simulink model "multi_ca_sim_1"  (R2020a)
settings: Solver=FixedStepAuto  StartTime=0.0  StopTime=23  FixedStep=0.01  MinStep=0.01  RelTol=1e-3
values from neighbouring files (symbols this model uses):
  ar_max = beta^2*omega/gamma/pi*0.999    (= 2.172825)    [SimulationSetup.m]
  beta = pi/tau_r    (= 3.14159265359)    [SimulationSetup.m]
  gamma = tau_r*beta + pi    (= 6.28318530718)    [SimulationSetup.m]
  Gamma = 10    [SimulationSetup.m]
  k = (gamma/beta)^2*(vo_max*psio_max) +0.1    (= 0.235)    [SimulationSetup.m]
  k_1 = 0.2    [SimulationSetup.m]
  k_2 = gamma^2/beta    (= 12.5663706144)    [SimulationSetup.m]
  k_delta = 1    [SimulationSetup.m]
  omega = r + (vr_max + vo_max)*pi/beta +0.1    (= 4.35)    [SimulationSetup.m]
  r = 2.0    (= 2)    [SimulationSetup.m]
  theta_0_1 = 0    [SimulationSetup.m]
  theta_0_2 = 0    [SimulationSetup.m]
  theta_0_3 = 0    [SimulationSetup.m]
  theta_a = pi/4    (= 0.785398163397)    [SimulationSetup.m]
  u_ca_max = 10    [SimulationSetup.m]
  u_tr_max = min(beta,beta^2*omega/(vr_max*gamma))    [SimulationSetup.m]
  vo_max = 0.75    [SimulationSetup.m]
  vr_max = 1.5    [SimulationSetup.m]
  vr_min = 1.0    (= 1)    [SimulationSetup.m]
  x_F_0_1 = -6    [SimulationSetup.m]
  x_F_0_2 = -4    [SimulationSetup.m]
  x_F_0_3 = -5    [SimulationSetup.m]
  y_F_0_1 = 0    [SimulationSetup.m]
  y_F_0_2 = -2    [SimulationSetup.m]
  y_F_0_3 = -4    [SimulationSetup.m]
libraries: cstblocks x3, dspmathops x3
(part 1 of 2)
settings Model: Creator=thiagomarinho  LastModifiedBy=tcy98
settings DataIOCC: ReturnWorkspaceOutputs=off
settings DebuggingCC: ArithmeticOperatorsInVariantConditions=warning
settings SFSimCC: CustomCodeUndefinedFunction=UseInterfaceOnly

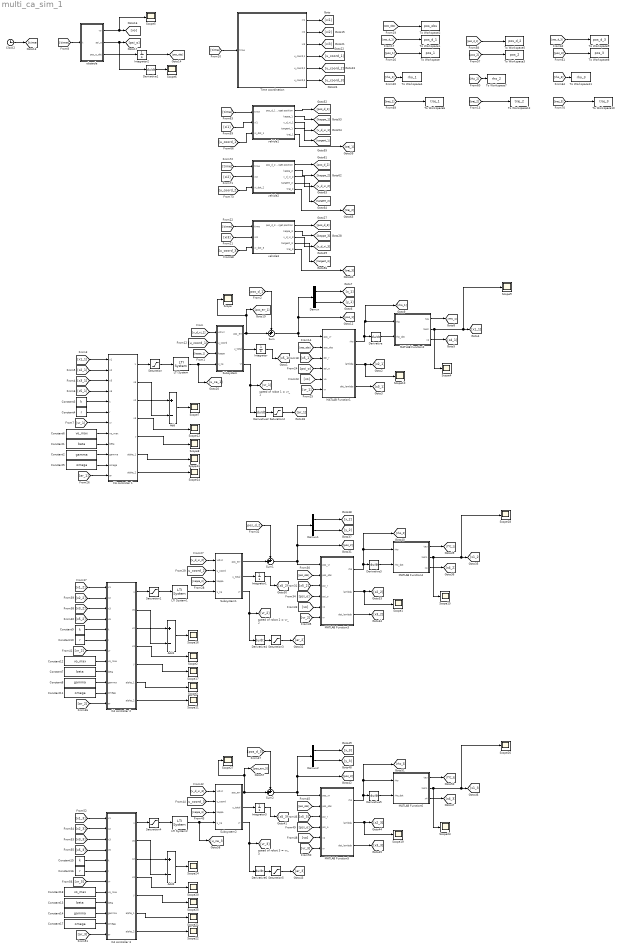
== system multi_ca_sim_1 ==
  Add : Sum  Inputs=+-
  Add1 : Sum  Inputs=+-
  Add2 : Sum  Inputs=+-
  CA controller 1 : MATLAB Function  TreatAsAtomicUnit=on
  CA controller 2 : MATLAB Function  TreatAsAtomicUnit=on
  CA controller 3 : MATLAB Function  TreatAsAtomicUnit=on
  Clock2 : Clock
  Constant1 : Constant  Value=beta
  Constant10 : Constant  Value=r
  Constant11 : Constant  Value=omega
  Constant12 : Constant  Value=vo_max
  Constant13 : Constant  Value=beta
  Constant14 : Constant  Value=gamma
  Constant15 : Constant  Value=k
  Constant16 : Constant  Value=r
  Constant17 : Constant  Value=omega
  Constant18 : Constant  Value=vo_max
  Constant2 : Constant  Value=gamma
  Constant3 : Constant  Value=k
  Constant4 : Constant  Value=r
  Constant5 : Constant  Value=omega
  Constant6 : Constant  Value=vo_max
  Constant7 : Constant  Value=beta
  Constant8 : Constant  Value=gamma
  Constant9 : Constant  Value=k
  Demux : Demux  Outputs=2
  Demux1 : Demux  Outputs=2
  Demux2 : Demux  Outputs=2
  Derivative{,1..6} (7 alike) : Derivative  CoefficientInTFapproximation=500
  Integrator : Integrator
  Integrator1 : Integrator
  Integrator2 : Integrator  InitialCondition=[0 0]'
  Integrator3 : Integrator
  LTI System : cstblocks/LTI System  sys=tf(1,[1 1])  IC=[]
  LTI System1 : cstblocks/LTI System  sys=tf(1,[1 1])  IC=[]
  LTI System2 : cstblocks/LTI System  sys=tf(1,[1 1])  IC=[]
  MATLAB Function1 : MATLAB Function  TreatAsAtomicUnit=on
  MATLAB Function2 : MATLAB Function  TreatAsAtomicUnit=on
  MATLAB Function3 : MATLAB Function  TreatAsAtomicUnit=on
  MATLAB Function4 : MATLAB Function  TreatAsAtomicUnit=on
  MATLAB Function5 : MATLAB Function  TreatAsAtomicUnit=on
  MATLAB Function6 : MATLAB Function  TreatAsAtomicUnit=on
  Saturation : Saturate  UpperLimit=u_ca_max  LowerLimit=-u_ca_max
  Saturation1 : Saturate  UpperLimit=u_ca_max  LowerLimit=-u_ca_max
  Saturation2 : Saturate  UpperLimit=ar_max  LowerLimit=-ar_max
  Saturation3 : Saturate  UpperLimit=ar_max  LowerLimit=-ar_max
  Saturation4 : Saturate  UpperLimit=u_ca_max  LowerLimit=-u_ca_max
  Saturation5 : Saturate  UpperLimit=ar_max  LowerLimit=-ar_max
  Scope{,1..27} (28 alike) : Scope
  Subsystem : Subsystem
  Subsystem1 : Subsystem
  Subsystem2 : Subsystem
  Sum : Sum  Inputs=++|
  Sum1 : Sum  Inputs=++|
  Sum2 : Sum  Inputs=++|
  Time coordination : Subsystem
  To Workspace : ToWorkspace  VariableName=pos_1  SaveFormat=Structure With Time  SampleTime=-1
  To Workspace1 : ToWorkspace  VariableName=pos_d_1  SaveFormat=Structure With Time  SampleTime=-1
  To Workspace10 : ToWorkspace  VariableName=traj_3  SaveFormat=Timeseries  SampleTime=-1
  To Workspace11 : ToWorkspace  VariableName=rho_3  SaveFormat=Timeseries  SampleTime=-1
  To Workspace12 : ToWorkspace  VariableName=traj_2  SaveFormat=Timeseries  SampleTime=-1
  To Workspace2 : ToWorkspace  VariableName=pos_obs  SaveFormat=Structure With Time  SampleTime=-1
  To Workspace3 : ToWorkspace  VariableName=pos_2  SaveFormat=Structure With Time  SampleTime=-1
  To Workspace4 : ToWorkspace  VariableName=rho_1  SaveFormat=Timeseries  SampleTime=-1
  To Workspace5 : ToWorkspace  VariableName=pos_d_2  SaveFormat=Structure With Time  SampleTime=-1
  To Workspace6 : ToWorkspace  VariableName=traj_1  SaveFormat=Timeseries  SampleTime=-1
  To Workspace7 : ToWorkspace  VariableName=rho_2  SaveFormat=Timeseries  SampleTime=-1
  To Workspace8 : ToWorkspace  VariableName=pos_3  SaveFormat=Structure With Time  SampleTime=-1
  To Workspace9 : ToWorkspace  VariableName=pos_d_3  SaveFormat=Structure With Time  SampleTime=-1
  obstacle : MATLAB Function  TreatAsAtomicUnit=on
  vehicle1 : Subsystem
  vehicle2 : Subsystem
  vehicle3 : Subsystem
  wires:
  obstacle/1(vo) -> Scope5/1, [vo]
  obstacle/2(psi_o) -> Derivative1/1, [psi_o]
  Integrator2/1 -> [pos_obs]
  obstacle/3(pos_o_dot) -> Integrator2/1
  Derivative1/1 -> Scope6/1
  [pos_obs] -> To Workspace2/1
  [pos_d_1] -> To Workspace1/1
  [v_d_xi_1] -> Subsystem/1(vd(xi))
  [kappa_1] -> Subsystem/3(kappa)
  [pos_d_1] -> Sum/1
  LTI System/1 -> [u_ca_1], Subsystem/4(u_ca)
  [pos_1] -> To Workspace/1
  MATLAB Function2/2(loom) -> Scope9/1, [x1_1], Scope4/1
  [vr_1] -> MATLAB Function1/6(vr)
  [x5_1] -> MATLAB Function1/3(psi_r)
  [vo] -> MATLAB Function1/5(vo)
  Demux/2 -> [y_1]
  MATLAB Function2/1(tau) -> [TTC_1]
  Derivative/1 -> MATLAB Function2/2(rho_dot)
  MATLAB Function2/3(x4) -> [x4_1]
  Demux/1 -> [x_1]
  MATLAB Function1/3(dot_lambda) -> [x3_1]
  [psi_o] -> MATLAB Function1/4(psi_o)
  MATLAB Function1/2(lambda) -> Scope10/1, [x2_1]
  [pos_obs] -> MATLAB Function1/2(pos_obs)
  MATLAB Function1/1(rho) -> [rho_1], MATLAB Function2/1(rho), Derivative/1
  CA controller 1/2(x5) -> Add/1
  CA controller 1/6(alpha_1) -> Scope13/1
  CA controller 1/5(y) -> Scope8/1
  [ar_1] -> CA controller 1/12(ar)
  [vr_1] -> CA controller 1/7(vr)
  CA controller 1/4(x3) -> Scope12/1
  CA controller 1/3(x2) -> Add/2
  Saturation/1 -> LTI System/1
  Constant5/1 -> CA controller 1/11(omega)
  Constant2/1 -> CA controller 1/10(gamma)
  CA controller 1/7(alpha_2) -> Scope14/1
  Constant1/1 -> CA controller 1/9(beta)
  Constant6/1 -> CA controller 1/8(vo_max)
  CA controller 1/1(u) -> Saturation/1
  Add/1 -> Scope7/1
  [x1_1] -> CA controller 1/1(x1)
  Constant3/1 -> CA controller 1/5(k)
  [x3_1] -> CA controller 1/3("x3 ")
  [x5_1] -> CA controller 1/4("x5 ")
  Constant4/1 -> CA controller 1/6(r)
  [x2_1] -> CA controller 1/2("x2 ")
  Subsystem/2(u_total) -> Integrator/1
  Integrator/1 -> [x5_1]
  Subsystem/3(vr) -> Derivative2/1, [vr_1]
  [rho_1] -> To Workspace4/1
  Saturation2/1 -> [ar_1]
  Derivative2/1 -> Saturation2/1
  Clock2/1 -> [time]
  [time] -> obstacle/1(t)
  [time] -> Time coordination/1(time)
  Sum/1 -> Demux/1, [pos_1], MATLAB Function1/1(pos_vr)
  Subsystem/1(pos_err) -> Sum/2, Scope/1, [pos_err_1]
  Time coordination/1(xi1) -> [xi1]
  Time coordination/2(xi2) -> [xi2]
  Time coordination/3(xi3) -> [xi3]
  Time coordination/4(u_coord,1) -> [u_coord_1]
  Time coordination/5(u_coord,2) -> [u_coord_2]
  Time coordination/6(u_coord,3) -> [u_coord_3]
  [u_coord_1] -> Subsystem/2(u_coord)
  [pos_d_2] -> Sum1/1
  Sum1/1 -> Demux1/1, [pos_2], MATLAB Function3/1(pos_vr)
  [x5_2] -> CA controller 2/4("x5 ")
  Constant10/1 -> CA controller 2/6(r)
  Constant7/1 -> CA controller 2/9(beta)
  Demux1/2 -> [y_2]
  [x5_2] -> MATLAB Function3/3(psi_r)
  Constant8/1 -> CA controller 2/10(gamma)
  Saturation1/1 -> LTI System1/1
  Constant12/1 -> CA controller 2/8(vo_max)
  [x2_2] -> CA controller 2/2("x2 ")
  Subsystem1/2(u_total) -> Integrator1/1
  CA controller 2/2(x5) -> Add1/1
  [pos_obs] -> MATLAB Function3/2(pos_obs)
  MATLAB Function3/3(dot_lambda) -> [x3_2]
  MATLAB Function3/2(lambda) -> Scope1/1, [x2_2]
  MATLAB Function3/1(rho) -> [rho_2], MATLAB Function4/1(rho), Derivative3/1
  CA controller 2/1(u) -> Saturation1/1
  [vr_2] -> CA controller 2/7(vr)
  [kappa_2] -> Subsystem1/3(kappa)
  [vo] -> MATLAB Function3/5(vo)
  [ar_2] -> CA controller 2/12(ar)
  Constant11/1 -> CA controller 2/11(omega)
  CA controller 2/5(y) -> Scope17/1
  [vr_2] -> MATLAB Function3/6(vr)
  MATLAB Function4/2(loom) -> Scope18/1, [x1_2], Scope15/1
  CA controller 2/3(x2) -> Add1/2
  Derivative3/1 -> MATLAB Function4/2(rho_dot)
  MATLAB Function4/1(tau) -> [TTC_2]
  MATLAB Function4/3(x4) -> [x4_2]
  Subsystem1/1(pos_err) -> Sum1/2
  Constant9/1 -> CA controller 2/5(k)
  [x3_2] -> CA controller 2/3("x3 ")
  Derivative4/1 -> Saturation3/1
  [x1_2] -> CA controller 2/1(x1)
  CA controller 2/7(alpha_2) -> Scope11/1
  Integrator1/1 -> [x5_2]
  Subsystem1/3(vr) -> Derivative4/1, [vr_2]
  [v_d_xi_2] -> Subsystem1/1(vd(xi))
  Add1/1 -> Scope16/1
  [psi_o] -> MATLAB Function3/4(psi_o)
  LTI System1/1 -> Subsystem1/4(u_ca)
  [u_coord_2] -> Subsystem1/2(u_coord)
  Saturation3/1 -> [ar_2]
  CA controller 2/6(alpha_1) -> Scope3/1
  CA controller 2/4(x3) -> Scope2/1
  Demux1/1 -> [x_2]
  [pos_d_3] -> Sum2/1
  Sum2/1 -> Demux2/1, [pos_3], MATLAB Function5/1(pos_vr)
  [x5_3] -> CA controller 3/4("x5 ")
  Constant16/1 -> CA controller 3/6(r)
  Constant13/1 -> CA controller 3/9(beta)
  Demux2/2 -> [y_3]
  [x5_3] -> MATLAB Function5/3(psi_r)
  Constant14/1 -> CA controller 3/10(gamma)
  Saturation4/1 -> LTI System2/1
  Constant18/1 -> CA controller 3/8(vo_max)
  [x2_3] -> CA controller 3/2("x2 ")
  Subsystem2/2(u_total) -> Integrator3/1
  CA controller 3/2(x5) -> Add2/1
  [pos_obs] -> MATLAB Function5/2(pos_obs)
  MATLAB Function5/3(dot_lambda) -> [x3_3]
  MATLAB Function5/2(lambda) -> Scope19/1, [x2_3]
  MATLAB Function5/1(rho) -> [rho_3], MATLAB Function6/1(rho), Derivative5/1
  CA controller 3/1(u) -> Saturation4/1
  [vr_3] -> CA controller 3/7(vr)
  [kappa_3] -> Subsystem2/3(kappa)
  [vo] -> MATLAB Function5/5(vo)
  [ar_3] -> CA controller 3/12(ar)
  Constant17/1 -> CA controller 3/11(omega)
  CA controller 3/5(y) -> Scope25/1
  [vr_3] -> MATLAB Function5/6(vr)
  MATLAB Function6/2(loom) -> Scope26/1, [x1_3], Scope23/1
  CA controller 3/3(x2) -> Add2/2
  Derivative5/1 -> MATLAB Function6/2(rho_dot)
  MATLAB Function6/1(tau) -> [TTC_3]
  MATLAB Function6/3(x4) -> [x4_3]
  Subsystem2/1(pos_err) -> Sum2/2, Scope27/1, [pos_err_3]
  Constant15/1 -> CA controller 3/5(k)
  [x3_3] -> CA controller 3/3("x3 ")
  Derivative6/1 -> Saturation5/1
  [x1_3] -> CA controller 3/1(x1)
  CA controller 3/7(alpha_2) -> Scope22/1
  Integrator3/1 -> [x5_3]
  Subsystem2/3(vr) -> Derivative6/1, [vr_3]
  [v_d_xi_3] -> Subsystem2/1(vd(xi))
  Add2/1 -> Scope24/1
  [psi_o] -> MATLAB Function5/4(psi_o)
  LTI System2/1 -> [u_ca_3], Subsystem2/4(u_ca)
  [u_coord_3] -> Subsystem2/2(u_coord)
  Saturation5/1 -> [ar_3]
  CA controller 3/6(alpha_1) -> Scope21/1
  CA controller 3/4(x3) -> Scope20/1
  Demux2/1 -> [x_3]
  [pos_2] -> To Workspace3/1
  [rho_2] -> To Workspace7/1
  [pos_d_2] -> To Workspace5/1
  [pos_3] -> To Workspace8/1
  [rho_3] -> To Workspace11/1
  [pos_d_3] -> To Workspace9/1
  vehicle1/4(tangent_1) -> [tangent_1]
  vehicle1/1(pos_d_1 = target position) -> [pos_d_1]
  [time] -> vehicle1/1(time)
  [u_coord_1] -> vehicle1/3(xi_dot_1)
  [xi1] -> vehicle1/2(xi1)
  vehicle1/3(v_d_xi_1) -> [v_d_xi_1]
  vehicle1/2(kappa_1) -> [kappa_1]
  [xi3] -> vehicle3/2(xi3)
  vehicle3/4(tangent_3) -> [tangent_3]
  vehicle3/3(v_d_xi_3) -> [v_d_xi_3]
  [u_coord_3] -> vehicle3/3(xi_dot_3)
  vehicle3/1(pos_d_3 = target position) -> [pos_d_3]
  vehicle3/2(kappa_3) -> [kappa_3]
  [time] -> vehicle3/1(time)
  vehicle1/5(traj_1) -> [traj_1]
  vehicle3/5(traj_3) -> [traj_3]
  [traj_1] -> To Workspace6/1
  [traj_3] -> To Workspace10/1
  vehicle2/4(tangent_2) -> [tangent_2]
  vehicle2/2(kappa_2) -> [kappa_2]
  vehicle2/5(traj_2) -> [traj_2]
  [xi2] -> vehicle2/2(xi2)
  [u_coord_2] -> vehicle2/3(xi_dot_2)
  vehicle2/3(v_d_xi_2) -> [v_d_xi_2]
  [time] -> vehicle2/1(time)
  vehicle2/1(pos_d_2 = target position) -> [pos_d_2]
  [traj_2] -> To Workspace12/1

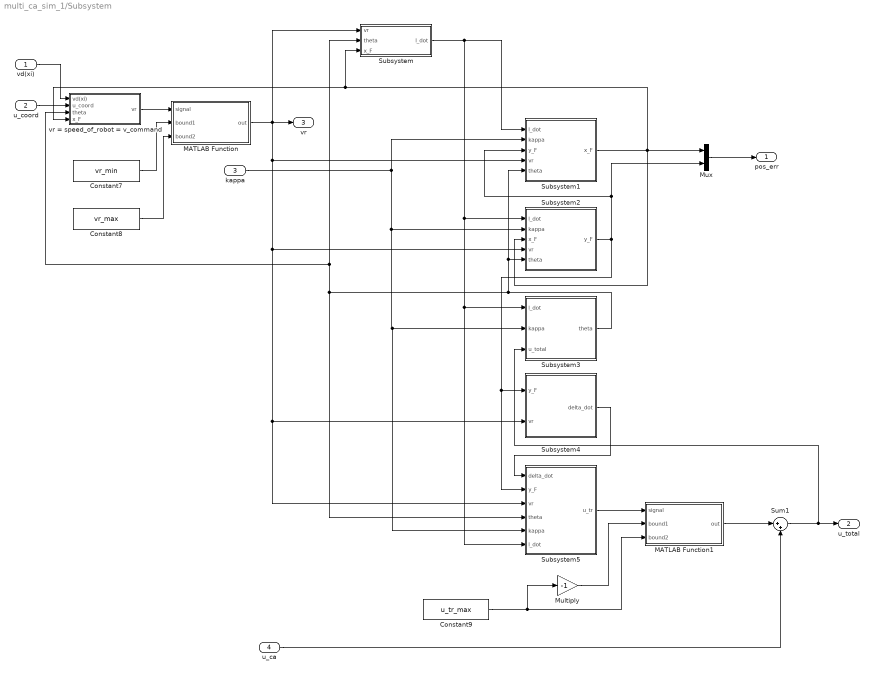
== system multi_ca_sim_1/Subsystem ==
  vd(xi) : Inport
  u_coord : Inport  Port=2
  kappa : Inport  Port=3
  u_ca : Inport  Port=4
  Constant7 : Constant  Value=vr_min
  Constant8 : Constant  Value=vr_max
  Constant9 : Constant  Value=u_tr_max
  MATLAB Function : MATLAB Function  TreatAsAtomicUnit=on
  MATLAB Function1 : MATLAB Function  TreatAsAtomicUnit=on
  Multiply : Gain  Gain=-1
  Mux : Mux  Inputs=2
  Subsystem : Subsystem
  Subsystem1 : Subsystem
  Subsystem2 : Subsystem
  Subsystem3 : Subsystem
  Subsystem4 : Subsystem
  Subsystem5 : Subsystem
  Sum1 : Sum  Inputs=|++
  vr = speed_of_robot = v_command : Subsystem
  pos_err : Outport  VectorParamsAs1DForOutWhenUnconnected=off
  u_total : Outport  Port=2  VectorParamsAs1DForOutWhenUnconnected=off
  vr : Outport  Port=3  VectorParamsAs1DForOutWhenUnconnected=off
  wires:
  Subsystem/1(l_dot) -> Subsystem1/1(l_dot), Subsystem5/6(l_dot), Subsystem3/1(l_dot), Subsystem2/1(l_dot)
  kappa/1 -> Subsystem5/5(kappa), Subsystem3/2(kappa), Subsystem2/2(kappa), Subsystem1/2(kappa)
  Subsystem2/1(y_F) -> Mux/2, Subsystem1/3(y_F), Subsystem5/2(y_F), Subsystem4/1(y_F)
  Subsystem1/1(x_F) -> Mux/1, vr = speed_of_robot = v_command/4(x_F), Subsystem/3(x_F), Subsystem2/3(x_F)
  Subsystem3/1(theta) -> vr = speed_of_robot = v_command/3(theta), Subsystem/2(theta), Subsystem5/4(theta), Subsystem1/5(theta), Subsystem2/5(theta)
  Subsystem4/1(delta_dot) -> Subsystem5/1(delta_dot)
  Mux/1 -> pos_err/1
  vd(xi)/1 -> vr = speed_of_robot = v_command/1(vd(xi))
  Sum1/1 -> Subsystem3/3(u_total), u_total/1
  u_ca/1 -> Sum1/2
  vr = speed_of_robot = v_command/1(vr) -> MATLAB Function/1(signal)
  MATLAB Function/1(out) -> Subsystem5/3(vr), Subsystem4/2(vr), Subsystem2/4(vr), Subsystem1/4(vr), Subsystem/1(vr), vr/1
  Constant7/1 -> MATLAB Function/2(bound1)
  Constant8/1 -> MATLAB Function/3(bound2)
  Subsystem5/1(u_tr) -> MATLAB Function1/1(signal)
  MATLAB Function1/1(out) -> Sum1/1
  Constant9/1 -> Multiply/1, MATLAB Function1/3(bound2)
  Multiply/1 -> MATLAB Function1/2(bound1)
  u_coord/1 -> vr = speed_of_robot = v_command/2(u_coord)

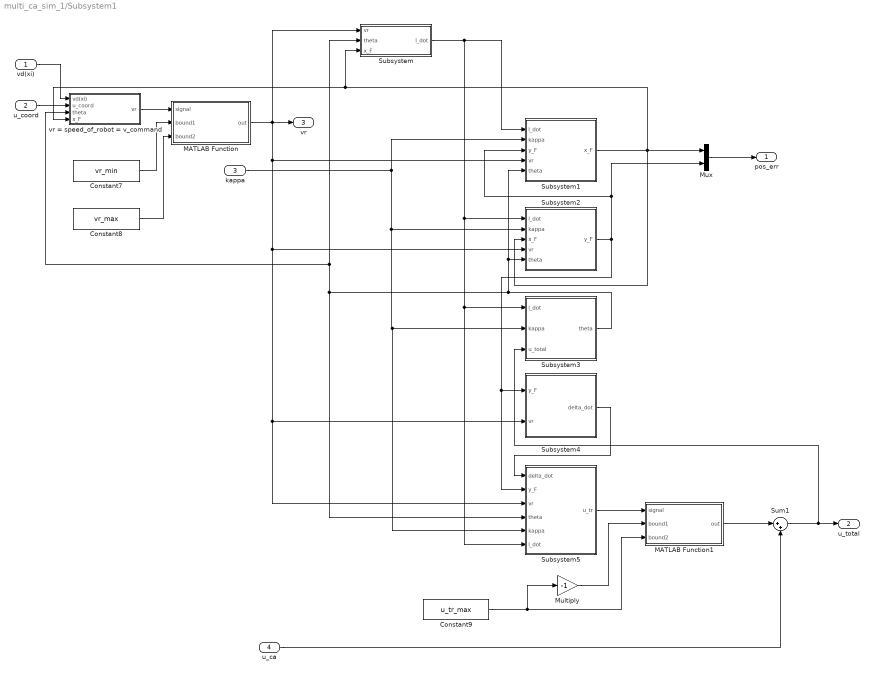
== system multi_ca_sim_1/Subsystem1 ==
  vd(xi) : Inport
  u_coord : Inport  Port=2
  kappa : Inport  Port=3
  u_ca : Inport  Port=4
  Constant7 : Constant  Value=vr_min
  Constant8 : Constant  Value=vr_max
  Constant9 : Constant  Value=u_tr_max
  MATLAB Function : MATLAB Function  TreatAsAtomicUnit=on
  MATLAB Function1 : MATLAB Function  TreatAsAtomicUnit=on
  Multiply : Gain  Gain=-1
  Mux : Mux  Inputs=2
  Subsystem : Subsystem
  Subsystem1 : Subsystem
  Subsystem2 : Subsystem
  Subsystem3 : Subsystem
  Subsystem4 : Subsystem
  Subsystem5 : Subsystem
  Sum1 : Sum  Inputs=|++
  vr = speed_of_robot = v_command : Subsystem
  pos_err : Outport  VectorParamsAs1DForOutWhenUnconnected=off
  u_total : Outport  Port=2  VectorParamsAs1DForOutWhenUnconnected=off
  vr : Outport  Port=3  VectorParamsAs1DForOutWhenUnconnected=off
  wires:
  Subsystem/1(l_dot) -> Subsystem1/1(l_dot), Subsystem5/6(l_dot), Subsystem3/1(l_dot), Subsystem2/1(l_dot)
  kappa/1 -> Subsystem5/5(kappa), Subsystem3/2(kappa), Subsystem2/2(kappa), Subsystem1/2(kappa)
  Subsystem2/1(y_F) -> Mux/2, Subsystem1/3(y_F), Subsystem5/2(y_F), Subsystem4/1(y_F)
  Subsystem1/1(x_F) -> Mux/1, vr = speed_of_robot = v_command/4(x_F), Subsystem/3(x_F), Subsystem2/3(x_F)
  Subsystem3/1(theta) -> vr = speed_of_robot = v_command/3(theta), Subsystem/2(theta), Subsystem5/4(theta), Subsystem1/5(theta), Subsystem2/5(theta)
  Subsystem4/1(delta_dot) -> Subsystem5/1(delta_dot)
  Mux/1 -> pos_err/1
  vd(xi)/1 -> vr = speed_of_robot = v_command/1(vd(xi))
  Sum1/1 -> Subsystem3/3(u_total), u_total/1
  u_ca/1 -> Sum1/2
  vr = speed_of_robot = v_command/1(vr) -> MATLAB Function/1(signal)
  MATLAB Function/1(out) -> Subsystem5/3(vr), Subsystem4/2(vr), Subsystem2/4(vr), Subsystem1/4(vr), Subsystem/1(vr), vr/1
  Constant7/1 -> MATLAB Function/2(bound1)
  Constant8/1 -> MATLAB Function/3(bound2)
  Subsystem5/1(u_tr) -> MATLAB Function1/1(signal)
  MATLAB Function1/1(out) -> Sum1/1
  Constant9/1 -> Multiply/1, MATLAB Function1/3(bound2)
  Multiply/1 -> MATLAB Function1/2(bound1)
  u_coord/1 -> vr = speed_of_robot = v_command/2(u_coord)

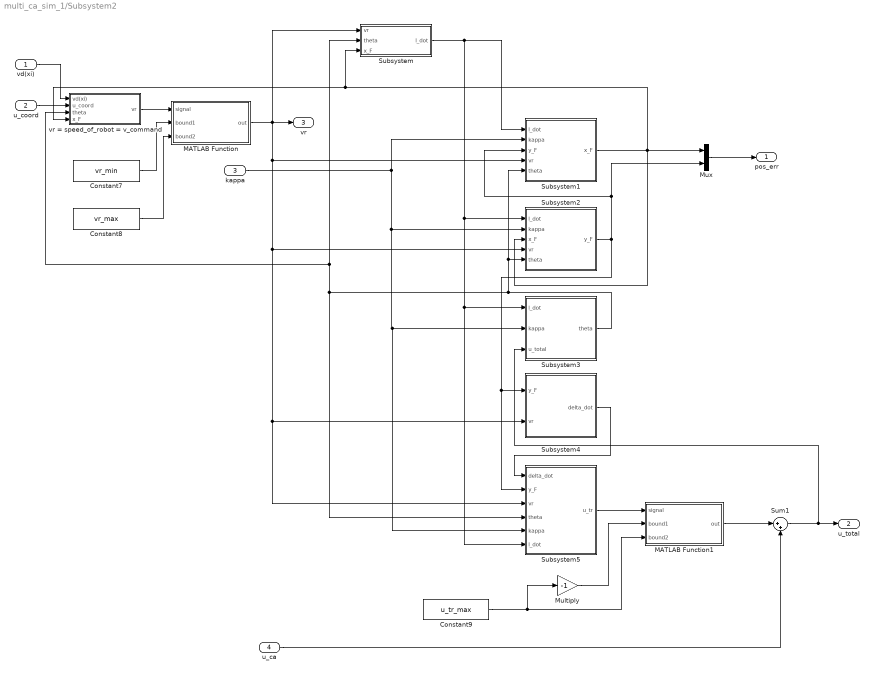
== system multi_ca_sim_1/Subsystem2 ==
  vd(xi) : Inport
  u_coord : Inport  Port=2
  kappa : Inport  Port=3
  u_ca : Inport  Port=4
  Constant7 : Constant  Value=vr_min
  Constant8 : Constant  Value=vr_max
  Constant9 : Constant  Value=u_tr_max
  MATLAB Function : MATLAB Function  TreatAsAtomicUnit=on
  MATLAB Function1 : MATLAB Function  TreatAsAtomicUnit=on
  Multiply : Gain  Gain=-1
  Mux : Mux  Inputs=2
  Subsystem : Subsystem
  Subsystem1 : Subsystem
  Subsystem2 : Subsystem
  Subsystem3 : Subsystem
  Subsystem4 : Subsystem
  Subsystem5 : Subsystem
  Sum1 : Sum  Inputs=|++
  vr = speed_of_robot = v_command : Subsystem
  pos_err : Outport  VectorParamsAs1DForOutWhenUnconnected=off
  u_total : Outport  Port=2  VectorParamsAs1DForOutWhenUnconnected=off
  vr : Outport  Port=3  VectorParamsAs1DForOutWhenUnconnected=off
  wires:
  Subsystem/1(l_dot) -> Subsystem1/1(l_dot), Subsystem5/6(l_dot), Subsystem3/1(l_dot), Subsystem2/1(l_dot)
  kappa/1 -> Subsystem5/5(kappa), Subsystem3/2(kappa), Subsystem2/2(kappa), Subsystem1/2(kappa)
  Subsystem2/1(y_F) -> Mux/2, Subsystem1/3(y_F), Subsystem5/2(y_F), Subsystem4/1(y_F)
  Subsystem1/1(x_F) -> Mux/1, vr = speed_of_robot = v_command/4(x_F), Subsystem/3(x_F), Subsystem2/3(x_F)
  Subsystem3/1(theta) -> vr = speed_of_robot = v_command/3(theta), Subsystem/2(theta), Subsystem5/4(theta), Subsystem1/5(theta), Subsystem2/5(theta)
  Subsystem4/1(delta_dot) -> Subsystem5/1(delta_dot)
  Mux/1 -> pos_err/1
  vd(xi)/1 -> vr = speed_of_robot = v_command/1(vd(xi))
  Sum1/1 -> Subsystem3/3(u_total), u_total/1
  u_ca/1 -> Sum1/2
  vr = speed_of_robot = v_command/1(vr) -> MATLAB Function/1(signal)
  MATLAB Function/1(out) -> Subsystem5/3(vr), Subsystem4/2(vr), Subsystem2/4(vr), Subsystem1/4(vr), Subsystem/1(vr), vr/1
  Constant7/1 -> MATLAB Function/2(bound1)
  Constant8/1 -> MATLAB Function/3(bound2)
  Subsystem5/1(u_tr) -> MATLAB Function1/1(signal)
  MATLAB Function1/1(out) -> Sum1/1
  Constant9/1 -> Multiply/1, MATLAB Function1/3(bound2)
  Multiply/1 -> MATLAB Function1/2(bound1)
  u_coord/1 -> vr = speed_of_robot = v_command/2(u_coord)

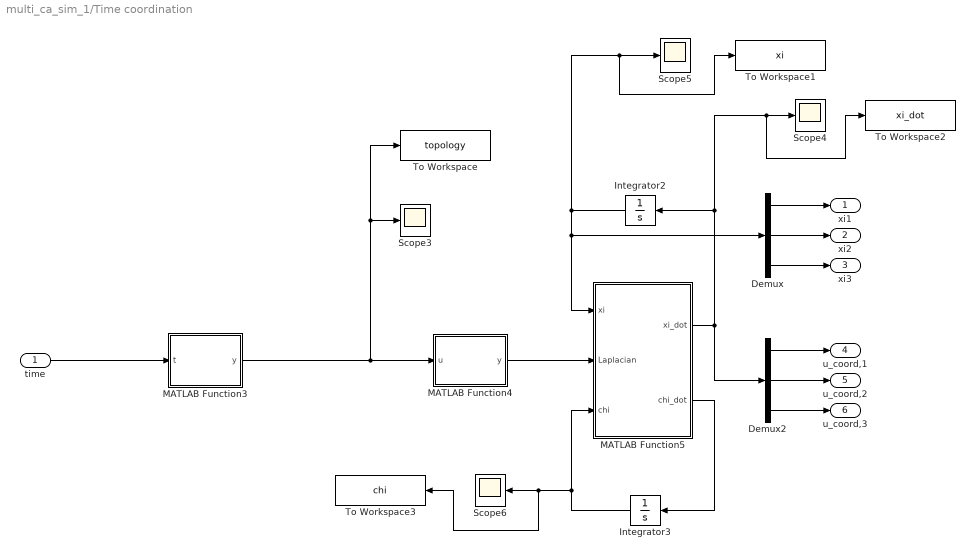
== system multi_ca_sim_1/Time coordination ==
  time : Inport
  Demux : Demux  Outputs=3
  Demux2 : Demux  Outputs=3
  Integrator2 : Integrator  InitialCondition=[0; 0; 0]
  Integrator3 : Integrator  InitialCondition=[1; 1]
  MATLAB Function3 : MATLAB Function  TreatAsAtomicUnit=on
  MATLAB Function4 : MATLAB Function  TreatAsAtomicUnit=on
  MATLAB Function5 : MATLAB Function  TreatAsAtomicUnit=on
  Scope{3..6} (4 alike) : Scope
  To Workspace : ToWorkspace  VariableName=topology  SaveFormat=Structure With Time  SampleTime=0.01
  To Workspace1 : ToWorkspace  VariableName=xi  SaveFormat=Structure With Time  SampleTime=0.01
  To Workspace2 : ToWorkspace  VariableName=xi_dot  SaveFormat=Structure With Time  SampleTime=0.01
  To Workspace3 : ToWorkspace  VariableName=chi  SaveFormat=Structure With Time  SampleTime=0.01
  xi1 : Outport  VectorParamsAs1DForOutWhenUnconnected=off
  xi2 : Outport  Port=2  VectorParamsAs1DForOutWhenUnconnected=off
  xi3 : Outport  Port=3  VectorParamsAs1DForOutWhenUnconnected=off
  u_coord,1 : Outport  Port=4  VectorParamsAs1DForOutWhenUnconnected=off
  u_coord,2 : Outport  Port=5  VectorParamsAs1DForOutWhenUnconnected=off
  u_coord,3 : Outport  Port=6  VectorParamsAs1DForOutWhenUnconnected=off
  wires:
  Demux/1 -> xi1/1
  Demux/2 -> xi2/1
  Demux/3 -> xi3/1
  Demux2/1 -> u_coord,1/1
  Demux2/2 -> u_coord,2/1
  Demux2/3 -> u_coord,3/1
  MATLAB Function3/1(y) -> MATLAB Function4/1(u), To Workspace/1, Scope3/1
  MATLAB Function4/1(y) -> MATLAB Function5/2(Laplacian)
  time/1 -> MATLAB Function3/1(t)
  MATLAB Function5/1(xi_dot) -> To Workspace2/1, Scope4/1, Integrator2/1, Demux2/1
  Integrator2/1 -> MATLAB Function5/1(xi), Demux/1, To Workspace1/1, Scope5/1
  Integrator3/1 -> To Workspace3/1, Scope6/1, MATLAB Function5/3(chi)
  MATLAB Function5/2(chi_dot) -> Integrator3/1

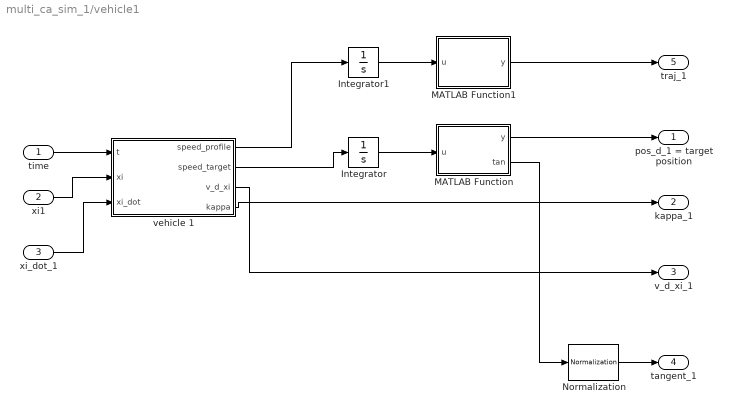
== system multi_ca_sim_1/vehicle1 ==
  time : Inport
  xi1 : Inport  Port=2
  xi_dot_1 : Inport  Port=3
  Integrator : Integrator
  Integrator1 : Integrator
  MATLAB Function : MATLAB Function  TreatAsAtomicUnit=on
  MATLAB Function1 : MATLAB Function  TreatAsAtomicUnit=on
  Normalization : dspmathops/Normalization  NormType=2-norm  Bias=1e-10  NormOver=Each column  Dimension=1  roundingMode=Floor  overflowMode=off  accumDataTypeStr=Inherit: Same as product output  accumLastDataTypeStr=Inherit: Same as product output  outputDataTypeStr=Inherit: Same as product output  outputMin=[]  outputMax=[]  outputLastDataTypeStr=Inherit: Same as product output
  vehicle 1 : MATLAB Function  TreatAsAtomicUnit=on
  pos_d_1 = target position : Outport  VectorParamsAs1DForOutWhenUnconnected=off
  kappa_1 : Outport  Port=2  VectorParamsAs1DForOutWhenUnconnected=off
  v_d_xi_1 : Outport  Port=3  VectorParamsAs1DForOutWhenUnconnected=off
  tangent_1 : Outport  Port=4  VectorParamsAs1DForOutWhenUnconnected=off
  traj_1 : Outport  Port=5  VectorParamsAs1DForOutWhenUnconnected=off
  wires:
  xi1/1 -> vehicle 1/2(xi)
  time/1 -> vehicle 1/1(t)
  vehicle 1/4(kappa) -> kappa_1/1
  Normalization/1 -> tangent_1/1
  vehicle 1/3(v_d_xi) -> v_d_xi_1/1
  vehicle 1/2(speed_target) -> Integrator/1
  Integrator/1 -> MATLAB Function/1(u)
  MATLAB Function/1(y) -> pos_d_1 = target position/1
  MATLAB Function/2(tan) -> Normalization/1
  xi_dot_1/1 -> vehicle 1/3(xi_dot)
  Integrator1/1 -> MATLAB Function1/1(u)
  vehicle 1/1(speed_profile) -> Integrator1/1
  MATLAB Function1/1(y) -> traj_1/1

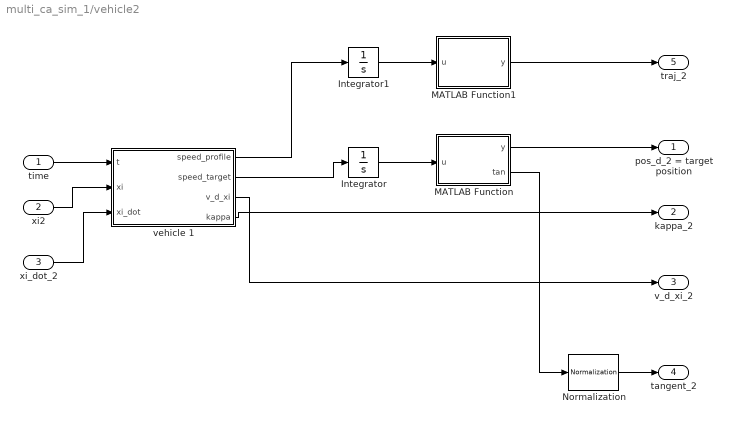
== system multi_ca_sim_1/vehicle2 ==
  time : Inport
  xi2 : Inport  Port=2
  xi_dot_2 : Inport  Port=3
  Integrator : Integrator
  Integrator1 : Integrator
  MATLAB Function : MATLAB Function  TreatAsAtomicUnit=on
  MATLAB Function1 : MATLAB Function  TreatAsAtomicUnit=on
  Normalization : dspmathops/Normalization  NormType=2-norm  Bias=1e-10  NormOver=Each column  Dimension=1  roundingMode=Floor  overflowMode=off  accumDataTypeStr=Inherit: Same as product output  accumLastDataTypeStr=Inherit: Same as product output  outputDataTypeStr=Inherit: Same as product output  outputMin=[]  outputMax=[]  outputLastDataTypeStr=Inherit: Same as product output
  vehicle 1 : MATLAB Function  TreatAsAtomicUnit=on
  pos_d_2 = target position : Outport  VectorParamsAs1DForOutWhenUnconnected=off
  kappa_2 : Outport  Port=2  VectorParamsAs1DForOutWhenUnconnected=off
  v_d_xi_2 : Outport  Port=3  VectorParamsAs1DForOutWhenUnconnected=off
  tangent_2 : Outport  Port=4  VectorParamsAs1DForOutWhenUnconnected=off
  traj_2 : Outport  Port=5  VectorParamsAs1DForOutWhenUnconnected=off
  wires:
  xi2/1 -> vehicle 1/2(xi)
  time/1 -> vehicle 1/1(t)
  vehicle 1/4(kappa) -> kappa_2/1
  vehicle 1/3(v_d_xi) -> v_d_xi_2/1
  Normalization/1 -> tangent_2/1
  Integrator/1 -> MATLAB Function/1(u)
  vehicle 1/2(speed_target) -> Integrator/1
  MATLAB Function/2(tan) -> Normalization/1
  MATLAB Function/1(y) -> pos_d_2 = target position/1
  xi_dot_2/1 -> vehicle 1/3(xi_dot)
  MATLAB Function1/1(y) -> traj_2/1
  Integrator1/1 -> MATLAB Function1/1(u)
  vehicle 1/1(speed_profile) -> Integrator1/1

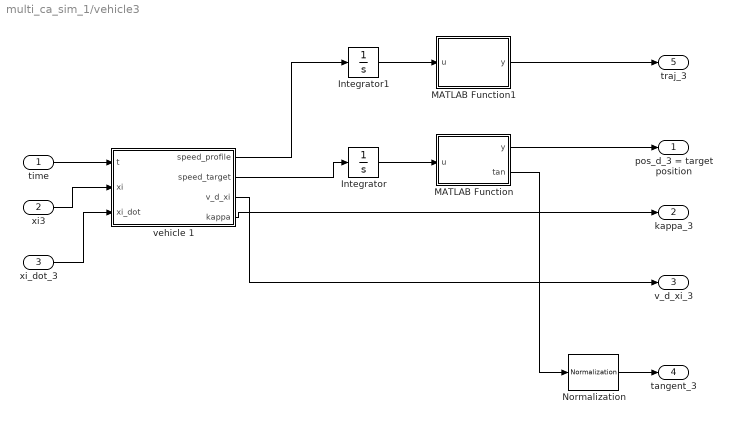
== system multi_ca_sim_1/vehicle3 ==
  time : Inport
  xi3 : Inport  Port=2
  xi_dot_3 : Inport  Port=3
  Integrator : Integrator
  Integrator1 : Integrator
  MATLAB Function : MATLAB Function  TreatAsAtomicUnit=on
  MATLAB Function1 : MATLAB Function  TreatAsAtomicUnit=on
  Normalization : dspmathops/Normalization  NormType=2-norm  Bias=1e-10  NormOver=Each column  Dimension=1  roundingMode=Floor  overflowMode=off  accumDataTypeStr=Inherit: Same as product output  accumLastDataTypeStr=Inherit: Same as product output  outputDataTypeStr=Inherit: Same as product output  outputMin=[]  outputMax=[]  outputLastDataTypeStr=Inherit: Same as product output
  vehicle 1 : MATLAB Function  TreatAsAtomicUnit=on
  pos_d_3 = target position : Outport  VectorParamsAs1DForOutWhenUnconnected=off
  kappa_3 : Outport  Port=2  VectorParamsAs1DForOutWhenUnconnected=off
  v_d_xi_3 : Outport  Port=3  VectorParamsAs1DForOutWhenUnconnected=off
  tangent_3 : Outport  Port=4  VectorParamsAs1DForOutWhenUnconnected=off
  traj_3 : Outport  Port=5  VectorParamsAs1DForOutWhenUnconnected=off
  wires:
  xi3/1 -> vehicle 1/2(xi)
  time/1 -> vehicle 1/1(t)
  vehicle 1/4(kappa) -> kappa_3/1
  vehicle 1/3(v_d_xi) -> v_d_xi_3/1
  Normalization/1 -> tangent_3/1
  Integrator/1 -> MATLAB Function/1(u)
  vehicle 1/2(speed_target) -> Integrator/1
  MATLAB Function/2(tan) -> Normalization/1
  MATLAB Function/1(y) -> pos_d_3 = target position/1
  xi_dot_3/1 -> vehicle 1/3(xi_dot)
  MATLAB Function1/1(y) -> traj_3/1
  Integrator1/1 -> MATLAB Function1/1(u)
  vehicle 1/1(speed_profile) -> Integrator1/1

== system multi_ca_sim_1/Subsystem/Subsystem ==
  vr : Inport
  theta : Inport  Port=2
  x_F : Inport  Port=3
  Cos : Trigonometry  Operator=cos
  Multiply : Gain  Gain=k_1
  Product : Product
  Sum : Sum  Inputs=|++
  l_dot : Outport  VectorParamsAs1DForOutWhenUnconnected=off
  wires:
  theta/1 -> Cos/1
  vr/1 -> Product/1
  Cos/1 -> Product/2
  Product/1 -> Sum/1
  x_F/1 -> Multiply/1
  Multiply/1 -> Sum/2
  Sum/1 -> l_dot/1

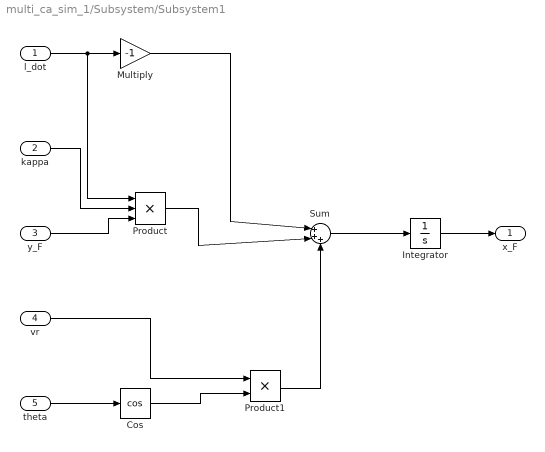
== system multi_ca_sim_1/Subsystem/Subsystem1 ==
  l_dot : Inport
  kappa : Inport  Port=2
  y_F : Inport  Port=3
  vr : Inport  Port=4
  theta : Inport  Port=5
  Cos : Trigonometry  Operator=cos
  Integrator : Integrator  InitialCondition=x_F_0_1
  Multiply : Gain  Gain=-1
  Product : Product  Inputs=3
  Product1 : Product
  Sum : Sum  Inputs=|+++
  x_F : Outport  VectorParamsAs1DForOutWhenUnconnected=off
  wires:
  l_dot/1 -> Product/1, Multiply/1
  Multiply/1 -> Sum/1
  kappa/1 -> Product/2
  y_F/1 -> Product/3
  Product/1 -> Sum/2
  theta/1 -> Cos/1
  vr/1 -> Product1/1
  Cos/1 -> Product1/2
  Product1/1 -> Sum/3
  Sum/1 -> Integrator/1
  Integrator/1 -> x_F/1

== system multi_ca_sim_1/Subsystem/Subsystem2 ==
  l_dot : Inport
  kappa : Inport  Port=2
  x_F : Inport  Port=3
  vr : Inport  Port=4
  theta : Inport  Port=5
  Integrator : Integrator  InitialCondition=y_F_0_1
  Multiply : Gain  Gain=-1
  Product : Product  Inputs=3
  Product1 : Product
  Sin : Trigonometry
  Sum : Sum  Inputs=|++
  y_F : Outport  VectorParamsAs1DForOutWhenUnconnected=off
  wires:
  l_dot/1 -> Product/1
  kappa/1 -> Product/2
  x_F/1 -> Product/3
  Product/1 -> Multiply/1
  theta/1 -> Sin/1
  vr/1 -> Product1/1
  Sin/1 -> Product1/2
  Sum/1 -> Integrator/1
  Integrator/1 -> y_F/1
  Multiply/1 -> Sum/1
  Product1/1 -> Sum/2

== system multi_ca_sim_1/Subsystem/Subsystem3 ==
  l_dot : Inport
  kappa : Inport  Port=2
  u_total : Inport  Port=3
  Integrator : Integrator  InitialCondition=theta_0_1
  Multiply : Gain  Gain=-1
  Product : Product
  Sum : Sum  Inputs=|++
  theta : Outport  VectorParamsAs1DForOutWhenUnconnected=off
  wires:
  l_dot/1 -> Product/1
  kappa/1 -> Product/2
  Product/1 -> Multiply/1
  Sum/1 -> Integrator/1
  Integrator/1 -> theta/1
  Multiply/1 -> Sum/1
  u_total/1 -> Sum/2

== system multi_ca_sim_1/Subsystem/Subsystem4 ==
  y_F : Inport
  vr : Inport  Port=2
  Constant : Constant  Value=k_delta
  Derivative : Derivative
  Multiply : Gain  Gain=-theta_a
  Product : Product  Inputs=3
  Tanh : Trigonometry  Operator=tanh
  delta_dot : Outport  VectorParamsAs1DForOutWhenUnconnected=off
  wires:
  Multiply/1 -> Derivative/1
  Derivative/1 -> delta_dot/1
  Constant/1 -> Product/1
  y_F/1 -> Product/2
  vr/1 -> Product/3
  Product/1 -> Tanh/1
  Tanh/1 -> Multiply/1

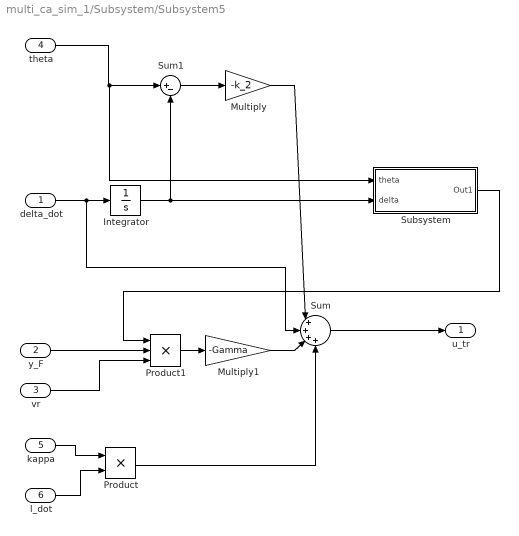
== system multi_ca_sim_1/Subsystem/Subsystem5 ==
  delta_dot : Inport
  y_F : Inport  Port=2
  vr : Inport  Port=3
  theta : Inport  Port=4
  kappa : Inport  Port=5
  l_dot : Inport  Port=6
  Integrator : Integrator
  Multiply : Gain  Gain=-k_2
  Multiply1 : Gain  Gain=-Gamma
  Product : Product
  Product1 : Product  Inputs=3
  Subsystem : Subsystem
  Sum : Sum  Inputs=|++++
  Sum1 : Sum  Inputs=|+-
  u_tr : Outport  VectorParamsAs1DForOutWhenUnconnected=off
  wires:
  Sum/1 -> u_tr/1
  kappa/1 -> Product/1
  l_dot/1 -> Product/2
  delta_dot/1 -> Sum/2, Integrator/1
  theta/1 -> Subsystem/1(theta), Sum1/1
  Integrator/1 -> Subsystem/2(delta), Sum1/2
  Sum1/1 -> Multiply/1
  Multiply/1 -> Sum/1
  y_F/1 -> Product1/2
  vr/1 -> Product1/3
  Product/1 -> Sum/4
  Product1/1 -> Multiply1/1
  Subsystem/1(Out1) -> Product1/1
  Multiply1/1 -> Sum/3

== system multi_ca_sim_1/Subsystem/vr = speed_of_robot = v_command ==
  vd(xi) : Inport
  u_coord : Inport  Port=2
  theta : Inport  Port=3
  x_F : Inport  Port=4
  Cos : Trigonometry  Operator=cos
  Divide : Product  Inputs=*/
  Multiply : Gain  Gain=k_1
  Product : Product
  Sum : Sum  Inputs=|+-
  vr : Outport  VectorParamsAs1DForOutWhenUnconnected=off
  wires:
  theta/1 -> Cos/1
  x_F/1 -> Multiply/1
  Multiply/1 -> Sum/2
  Sum/1 -> Divide/1
  Divide/1 -> vr/1
  Cos/1 -> Divide/2
  u_coord/1 -> Product/2
  Product/1 -> Sum/1
  vd(xi)/1 -> Product/1

== system multi_ca_sim_1/Subsystem1/Subsystem ==
  vr : Inport
  theta : Inport  Port=2
  x_F : Inport  Port=3
  Cos : Trigonometry  Operator=cos
  Multiply : Gain  Gain=k_1
  Product : Product
  Sum : Sum  Inputs=|++
  l_dot : Outport  VectorParamsAs1DForOutWhenUnconnected=off
  wires:
  theta/1 -> Cos/1
  vr/1 -> Product/1
  Cos/1 -> Product/2
  Product/1 -> Sum/1
  x_F/1 -> Multiply/1
  Multiply/1 -> Sum/2
  Sum/1 -> l_dot/1

== system multi_ca_sim_1/Subsystem1/Subsystem1 ==
  l_dot : Inport
  kappa : Inport  Port=2
  y_F : Inport  Port=3
  vr : Inport  Port=4
  theta : Inport  Port=5
  Cos : Trigonometry  Operator=cos
  Integrator : Integrator  InitialCondition=x_F_0_2
  Multiply : Gain  Gain=-1
  Product : Product  Inputs=3
  Product1 : Product
  Sum : Sum  Inputs=|+++
  x_F : Outport  VectorParamsAs1DForOutWhenUnconnected=off
  wires:
  l_dot/1 -> Product/1, Multiply/1
  Multiply/1 -> Sum/1
  kappa/1 -> Product/2
  y_F/1 -> Product/3
  Product/1 -> Sum/2
  theta/1 -> Cos/1
  vr/1 -> Product1/1
  Cos/1 -> Product1/2
  Product1/1 -> Sum/3
  Sum/1 -> Integrator/1
  Integrator/1 -> x_F/1

== system multi_ca_sim_1/Subsystem1/Subsystem2 ==
  l_dot : Inport
  kappa : Inport  Port=2
  x_F : Inport  Port=3
  vr : Inport  Port=4
  theta : Inport  Port=5
  Integrator : Integrator  InitialCondition=y_F_0_2
  Multiply : Gain  Gain=-1
  Product : Product  Inputs=3
  Product1 : Product
  Sin : Trigonometry
  Sum : Sum  Inputs=|++
  y_F : Outport  VectorParamsAs1DForOutWhenUnconnected=off
  wires:
  l_dot/1 -> Product/1
  kappa/1 -> Product/2
  x_F/1 -> Product/3
  Product/1 -> Multiply/1
  theta/1 -> Sin/1
  vr/1 -> Product1/1
  Sin/1 -> Product1/2
  Sum/1 -> Integrator/1
  Integrator/1 -> y_F/1
  Multiply/1 -> Sum/1
  Product1/1 -> Sum/2

== system multi_ca_sim_1/Subsystem1/Subsystem3 ==
  l_dot : Inport
  kappa : Inport  Port=2
  u_total : Inport  Port=3
  Integrator : Integrator  InitialCondition=theta_0_2
  Multiply : Gain  Gain=-1
  Product : Product
  Sum : Sum  Inputs=|++
  theta : Outport  VectorParamsAs1DForOutWhenUnconnected=off
  wires:
  l_dot/1 -> Product/1
  kappa/1 -> Product/2
  Product/1 -> Multiply/1
  Sum/1 -> Integrator/1
  Integrator/1 -> theta/1
  Multiply/1 -> Sum/1
  u_total/1 -> Sum/2

== system multi_ca_sim_1/Subsystem1/Subsystem4 ==
  y_F : Inport
  vr : Inport  Port=2
  Constant : Constant  Value=k_delta
  Derivative : Derivative
  Multiply : Gain  Gain=-theta_a
  Product : Product  Inputs=3
  Tanh : Trigonometry  Operator=tanh
  delta_dot : Outport  VectorParamsAs1DForOutWhenUnconnected=off
  wires:
  Multiply/1 -> Derivative/1
  Derivative/1 -> delta_dot/1
  Constant/1 -> Product/1
  y_F/1 -> Product/2
  vr/1 -> Product/3
  Product/1 -> Tanh/1
  Tanh/1 -> Multiply/1

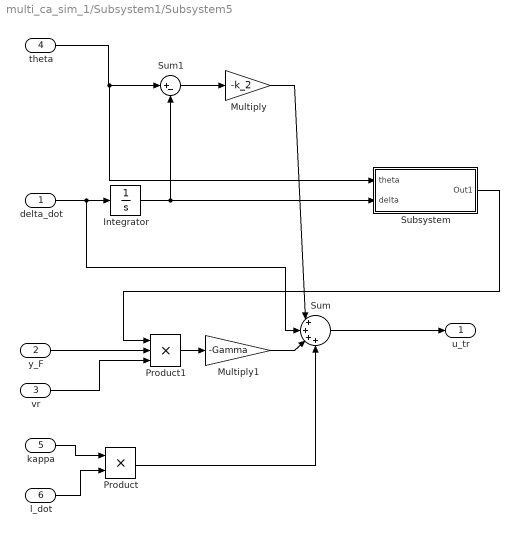
== system multi_ca_sim_1/Subsystem1/Subsystem5 ==
  delta_dot : Inport
  y_F : Inport  Port=2
  vr : Inport  Port=3
  theta : Inport  Port=4
  kappa : Inport  Port=5
  l_dot : Inport  Port=6
  Integrator : Integrator
  Multiply : Gain  Gain=-k_2
  Multiply1 : Gain  Gain=-Gamma
  Product : Product
  Product1 : Product  Inputs=3
  Subsystem : Subsystem
  Sum : Sum  Inputs=|++++
  Sum1 : Sum  Inputs=|+-
  u_tr : Outport  VectorParamsAs1DForOutWhenUnconnected=off
  wires:
  Sum/1 -> u_tr/1
  kappa/1 -> Product/1
  l_dot/1 -> Product/2
  delta_dot/1 -> Sum/2, Integrator/1
  theta/1 -> Subsystem/1(theta), Sum1/1
  Integrator/1 -> Subsystem/2(delta), Sum1/2
  Sum1/1 -> Multiply/1
  Multiply/1 -> Sum/1
  y_F/1 -> Product1/2
  vr/1 -> Product1/3
  Product/1 -> Sum/4
  Product1/1 -> Multiply1/1
  Subsystem/1(Out1) -> Product1/1
  Multiply1/1 -> Sum/3

== system multi_ca_sim_1/Subsystem1/vr = speed_of_robot = v_command ==
  vd(xi) : Inport
  u_coord : Inport  Port=2
  theta : Inport  Port=3
  x_F : Inport  Port=4
  Cos : Trigonometry  Operator=cos
  Divide : Product  Inputs=*/
  Multiply : Gain  Gain=k_1
  Product : Product
  Sum : Sum  Inputs=|+-
  vr : Outport  VectorParamsAs1DForOutWhenUnconnected=off
  wires:
  theta/1 -> Cos/1
  x_F/1 -> Multiply/1
  Multiply/1 -> Sum/2
  Sum/1 -> Divide/1
  Divide/1 -> vr/1
  Cos/1 -> Divide/2
  u_coord/1 -> Product/2
  Product/1 -> Sum/1
  vd(xi)/1 -> Product/1

== system multi_ca_sim_1/Subsystem2/Subsystem ==
  vr : Inport
  theta : Inport  Port=2
  x_F : Inport  Port=3
  Cos : Trigonometry  Operator=cos
  Multiply : Gain  Gain=k_1
  Product : Product
  Sum : Sum  Inputs=|++
  l_dot : Outport  VectorParamsAs1DForOutWhenUnconnected=off
  wires:
  theta/1 -> Cos/1
  vr/1 -> Product/1
  Cos/1 -> Product/2
  Product/1 -> Sum/1
  x_F/1 -> Multiply/1
  Multiply/1 -> Sum/2
  Sum/1 -> l_dot/1

== system multi_ca_sim_1/Subsystem2/Subsystem1 ==
  l_dot : Inport
  kappa : Inport  Port=2
  y_F : Inport  Port=3
  vr : Inport  Port=4
  theta : Inport  Port=5
  Cos : Trigonometry  Operator=cos
  Integrator : Integrator  InitialCondition=x_F_0_3
  Multiply : Gain  Gain=-1
  Product : Product  Inputs=3
  Product1 : Product
  Sum : Sum  Inputs=|+++
  x_F : Outport  VectorParamsAs1DForOutWhenUnconnected=off
  wires:
  l_dot/1 -> Product/1, Multiply/1
  Multiply/1 -> Sum/1
  kappa/1 -> Product/2
  y_F/1 -> Product/3
  Product/1 -> Sum/2
  theta/1 -> Cos/1
  vr/1 -> Product1/1
  Cos/1 -> Product1/2
  Product1/1 -> Sum/3
  Sum/1 -> Integrator/1
  Integrator/1 -> x_F/1

== system multi_ca_sim_1/Subsystem2/Subsystem2 ==
  l_dot : Inport
  kappa : Inport  Port=2
  x_F : Inport  Port=3
  vr : Inport  Port=4
  theta : Inport  Port=5
  Integrator : Integrator  InitialCondition=y_F_0_3
  Multiply : Gain  Gain=-1
  Product : Product  Inputs=3
  Product1 : Product
  Sin : Trigonometry
  Sum : Sum  Inputs=|++
  y_F : Outport  VectorParamsAs1DForOutWhenUnconnected=off
  wires:
  l_dot/1 -> Product/1
  kappa/1 -> Product/2
  x_F/1 -> Product/3
  Product/1 -> Multiply/1
  theta/1 -> Sin/1
  vr/1 -> Product1/1
  Sin/1 -> Product1/2
  Sum/1 -> Integrator/1
  Integrator/1 -> y_F/1
  Multiply/1 -> Sum/1
  Product1/1 -> Sum/2

== system multi_ca_sim_1/Subsystem2/Subsystem3 ==
  l_dot : Inport
  kappa : Inport  Port=2
  u_total : Inport  Port=3
  Integrator : Integrator  InitialCondition=theta_0_3
  Multiply : Gain  Gain=-1
  Product : Product
  Sum : Sum  Inputs=|++
  theta : Outport  VectorParamsAs1DForOutWhenUnconnected=off
  wires:
  l_dot/1 -> Product/1
  kappa/1 -> Product/2
  Product/1 -> Multiply/1
  Sum/1 -> Integrator/1
  Integrator/1 -> theta/1
  Multiply/1 -> Sum/1
  u_total/1 -> Sum/2

== system multi_ca_sim_1/Subsystem2/Subsystem4 ==
  y_F : Inport
  vr : Inport  Port=2
  Constant : Constant  Value=k_delta
  Derivative : Derivative
  Multiply : Gain  Gain=-theta_a
  Product : Product  Inputs=3
  Tanh : Trigonometry  Operator=tanh
  delta_dot : Outport  VectorParamsAs1DForOutWhenUnconnected=off
  wires:
  Multiply/1 -> Derivative/1
  Derivative/1 -> delta_dot/1
  Constant/1 -> Product/1
  y_F/1 -> Product/2
  vr/1 -> Product/3
  Product/1 -> Tanh/1
  Tanh/1 -> Multiply/1

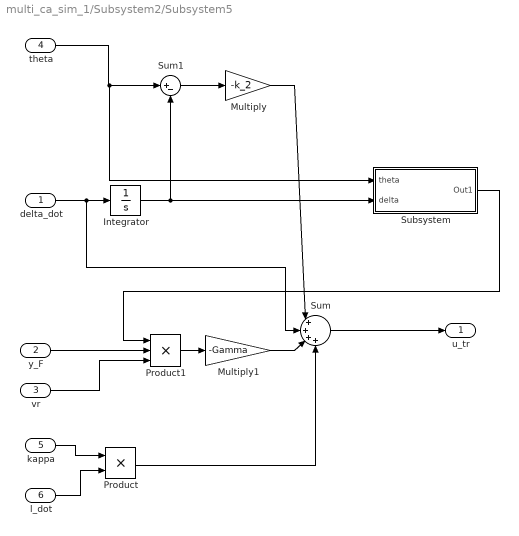
== system multi_ca_sim_1/Subsystem2/Subsystem5 ==
  delta_dot : Inport
  y_F : Inport  Port=2
  vr : Inport  Port=3
  theta : Inport  Port=4
  kappa : Inport  Port=5
  l_dot : Inport  Port=6
  Integrator : Integrator
  Multiply : Gain  Gain=-k_2
  Multiply1 : Gain  Gain=-Gamma
  Product : Product
  Product1 : Product  Inputs=3
  Subsystem : Subsystem
  Sum : Sum  Inputs=|++++
  Sum1 : Sum  Inputs=|+-
  u_tr : Outport  VectorParamsAs1DForOutWhenUnconnected=off
  wires:
  Sum/1 -> u_tr/1
  kappa/1 -> Product/1
  l_dot/1 -> Product/2
  delta_dot/1 -> Sum/2, Integrator/1
  theta/1 -> Subsystem/1(theta), Sum1/1
  Integrator/1 -> Subsystem/2(delta), Sum1/2
  Sum1/1 -> Multiply/1
  Multiply/1 -> Sum/1
  y_F/1 -> Product1/2
  vr/1 -> Product1/3
  Product/1 -> Sum/4
  Product1/1 -> Multiply1/1
  Subsystem/1(Out1) -> Product1/1
  Multiply1/1 -> Sum/3

== system multi_ca_sim_1/Subsystem2/vr = speed_of_robot = v_command ==
  vd(xi) : Inport
  u_coord : Inport  Port=2
  theta : Inport  Port=3
  x_F : Inport  Port=4
  Cos : Trigonometry  Operator=cos
  Divide : Product  Inputs=*/
  Multiply : Gain  Gain=k_1
  Product : Product
  Sum : Sum  Inputs=|+-
  vr : Outport  VectorParamsAs1DForOutWhenUnconnected=off
  wires:
  theta/1 -> Cos/1
  x_F/1 -> Multiply/1
  Multiply/1 -> Sum/2
  Sum/1 -> Divide/1
  Divide/1 -> vr/1
  Cos/1 -> Divide/2
  u_coord/1 -> Product/2
  Product/1 -> Sum/1
  vd(xi)/1 -> Product/1

== system multi_ca_sim_1/Subsystem/Subsystem5/Subsystem ==
  theta : Inport
  delta : Inport  Port=2
  MATLAB Function : MATLAB Function  TreatAsAtomicUnit=on
  Out1 : Outport  VectorParamsAs1DForOutWhenUnconnected=off
  wires:
  theta/1 -> MATLAB Function/1(theta)
  delta/1 -> MATLAB Function/2(delta)
  MATLAB Function/1(y) -> Out1/1

== system multi_ca_sim_1/Subsystem1/Subsystem5/Subsystem ==
  theta : Inport
  delta : Inport  Port=2
  MATLAB Function : MATLAB Function  TreatAsAtomicUnit=on
  Out1 : Outport  VectorParamsAs1DForOutWhenUnconnected=off
  wires:
  theta/1 -> MATLAB Function/1(theta)
  delta/1 -> MATLAB Function/2(delta)
  MATLAB Function/1(y) -> Out1/1

== system multi_ca_sim_1/Subsystem2/Subsystem5/Subsystem ==
  theta : Inport
  delta : Inport  Port=2
  MATLAB Function : MATLAB Function  TreatAsAtomicUnit=on
  Out1 : Outport  VectorParamsAs1DForOutWhenUnconnected=off
  wires:
  theta/1 -> MATLAB Function/1(theta)
  delta/1 -> MATLAB Function/2(delta)
  MATLAB Function/1(y) -> Out1/1

== matlab function multi_ca_sim_1/Subsystem/MATLAB Function1 ==
  data: signal input; out output; bound1 input; bound2 input
function out = saturate(signal,bound1,bound2)
            out = min(max(bound1,signal),bound2);

== matlab function multi_ca_sim_1/obstacle ==
  data: t input; vo output; psi_o output; pos_o_dot output
function [vo, psi_o, pos_o_dot] = fcn(t)
vo=0;%-1.5/3;
psi_o = t/pi/4/2 - pi/4 ;
x_dot = -vo*sin(-psi_o);
y_dot = vo*cos(-psi_o);
pos_o_dot = [x_dot ; y_dot];

== matlab function multi_ca_sim_1/Time coordination/MATLAB Function4 ==
  data: u input; y output
function y = fcn(u)

y=zeros(3,3);

switch u
    case 1
        y=[0 0 0; 0 0 0; 0 0 0];
    case 2
        y=[0 0 0; 0 1 -1; 0 -1 1];
    case 3
        y=[1 -1 0; -1 1 0; 0 0 0];
    case 4
        y=[1 0 -1; 0 0 0; -1 0 1];
    case 5
        y=[1 0 -1; -1 1 0; 0 -1 1];
    case 6
        y=[1 -1 0; 0 1 -1; -1 0 1];
    case 7
        y=[1 0 -1; 0 1 -1; -1 -1 2];
    case 8
        y=[1 -1 0; -1 2 -1; 0 -1 1];
    case 9
        y=[2 -1 -1; -1 1 0; -1 0 1];
    case 10
        y=[2 -1 -1; -1 2 -1; -1 -1 2];
end

% switch u
%     case 1
%         y=[0 0 0; 0 1 -1; 0 -1 1];
%     case 2
%         y=[1 -1 0; -1 1 0; 0 0 0];
%     case 3
%         y=[1 0 -1; 0 0 0; -1 0 1];
% end

% switch u
%     case 1
%         y(1,2)=0; y(1,3)=0; y(2,3)=0;
%     case 2
%         y(1,2)=1; y(1,3)=0; y(2,3)=0;
%     case 3
%         y(1,2)=0; y(1,3)=1; y(2,3)=0;
%     case 4
%         y(1,2)=0; y(1,3)=0; y(2,3)=1;
%     case 5
%         y(1,2)=1; y(1,3)=1; y(2,3)=0;
%     case 6
%         y(1,2)=1; y(1,3)=0; y(2,3)=1;
%     case 7
%         y(1,2)=0; y(1,3)=1; y(2,3)=1;
%     case 8
%         y(1,2)=1; y(1,3)=1; y(2,3)=1;
% end
% 
% y(2,1)=y(1,2);
% y(3,1)=y(1,3);
% y(3,2)=y(2,3);
% y(1,1)=-y(1,2)-y(1,3);
% y(2,2)=-y(2,1)-y(2,3);
% y(3,3)=-y(3,1)-y(3,2);
% y=-y;

== matlab function multi_ca_sim_1/vehicle3/MATLAB Function ==
  data: u input; y output; tan output
function [y,tan] = fcn(u)
theta = u/(2*1.5*4*pi);
y = [cos(theta) -sin(theta); sin(theta) cos(theta)]*[2*1.5*4*pi; 0];%*[5+6*pi*sin(pi/4)-6*pi*sin(1.2*pi/4)-0.5 15+6*pi*cos(pi/4)-6*pi*cos(1.2*pi/4)]';
tan = [-y(2); y(1)];

== matlab function multi_ca_sim_1/vehicle3/vehicle 1 ==
  data: speed_profile output; speed_target output; v_d_xi output; kappa output; t input; xi input; xi_dot input
function [speed_profile, speed_target, v_d_xi, kappa] = fcn(t,xi,xi_dot)
% vd=1.5;
% psi_d = t/pi/4 - pi/4;
% x_dot = 1.5*cos(psi_d);
% y_dot = 1.5*sin(psi_d);

%trajectory and speed profile
% x_dot = 1*1.5*cos(t/pi/4 - 1.2*pi/4);
% y_dot = 0.9*1.5*sin(t/pi/4 - 1.2*pi/4);
speed_profile = 2*1.5;

%v_d(xi)
v_d_xi=2*1.5;
% v_d_xi=sqrt((0.9*1.5*cos(xi/pi/4 - 1.2*pi/4))^2+(0.9*1.5*sin(xi/pi/4 - 1.2*pi/4))^2);

%speed of target
speed_target = xi_dot*2*1.5;

%culvature
r=2*1.5*4*pi;
kappa=1/r;

== matlab function multi_ca_sim_1/vehicle1/MATLAB Function1 ==
  data: u input; y output
function y = fcn(u)
theta = u/(1*1.5*4*pi);
y = [cos(theta) -sin(theta); sin(theta) cos(theta)]*[1*1.5*4*pi; 0];%*[5+6*pi*sin(pi/4)-6*pi*sin(1.2*pi/4)-0.5 15+6*pi*cos(pi/4)-6*pi*cos(1.2*pi/4)]';

== matlab function multi_ca_sim_1/vehicle3/MATLAB Function1 ==
  data: u input; y output
function y = fcn(u)
theta = u/(2*1.5*4*pi);
y = [cos(theta) -sin(theta); sin(theta) cos(theta)]*[2*1.5*4*pi; 0];%*[5+6*pi*sin(pi/4)-6*pi*sin(1.2*pi/4)-0.5 15+6*pi*cos(pi/4)-6*pi*cos(1.2*pi/4)]';

== matlab function multi_ca_sim_1/CA controller 2 ==
  data: u output; x1 input; x2 input; x3 input; x5 input; k input; r input; vr input; vo_max input; beta input; gamma input; omega input; ar input; x5 output; x2 output; x3 output; y output; alpha_1 output; alpha_2 output
function [u, x5, x2, x3,y, alpha_1, alpha_2]  = fcn(x1, x2 ,x3, x5, k, r, vr, vo_max,beta, gamma,omega, ar)


x6 = vr;

delta_t = ( pi - abs(wrapToPi_custom(x5-x2)))/(beta);

alpha_2 = -2*beta*omega*x1/(x6+vo_max);
alpha_1 = (k*x1^2 +  x6*max(0,-x3*sin(x5-x2)) -min(0, -ar*cos(x5-x2)) ) /(r + (x6 + vo_max )*delta_t);

 u =  sign_custom(wrapToPi_custom(x5-x2))*(gamma^2/beta*(x1^2  +alpha_1 ) +  alpha_2) + x3  ;
y = sign_custom(wrapToPi_custom(x5-x2));

if x1 >= 0
    u=0;
end

function y = sign_custom(x)

if x >= 0
    y = 1;
else
    y = -1;
end

function lambda = wrapTo2Pi_custom(lambda)
%wrapTo2Pi Wrap angle in radians to [0 2*pi]
%
%   lambdaWrapped = wrapTo2Pi(LAMBDA) wraps angles in LAMBDA, in radians,
%   to the interval [0 2*pi] such that zero maps to zero and 2*pi maps
%   to 2*pi. (In general, positive multiples of 2*pi map to 2*pi and
%   negative multiples of 2*pi map to zero.)
%
%   See also wrapToPi, wrapTo180, wrapTo360.

% Copyright 2007-2008 The MathWorks, Inc.

positiveInput = (lambda > 0);
lambda = mod(lambda, 2*pi);
lambda((lambda == 0) & positiveInput) = 2*pi;

function lambda = wrapToPi_custom(lambda)
%wrapToPi Wrap angle in radians to [-pi pi]
%
%   lambdaWrapped = wrapToPi(LAMBDA) wraps angles in LAMBDA, in radians,
%   to the interval [-pi pi] such that pi maps to pi and -pi maps to
%   -pi.  (In general, odd, positive multiples of pi map to pi and odd,
%   negative multiples of pi map to -pi.)
%
%   See also wrapTo2Pi, wrapTo180, wrapTo360.

% Copyright 2007-2008 The MathWorks, Inc.

q = (lambda < -pi) | (pi < lambda);
lambda(q) = wrapTo2Pi_custom(lambda(q) + pi) - pi;

== matlab function multi_ca_sim_1/MATLAB Function3 ==
  data: rho output; pos_vr input; lambda output; pos_obs input; psi_r input; psi_o input; vo input; vr input; dot_lambda output
function [rho, lambda, dot_lambda] = fcn(pos_vr, pos_obs, psi_r, psi_o, vo, vr)

lambda_vector = pos_obs-pos_vr;
rho = norm(lambda_vector,2);
lambda = atan2(lambda_vector(2), lambda_vector(1) );
dot_lambda = 1/rho*(vo*sin(psi_o - lambda) - vr*sin(psi_r - lambda));

== matlab function multi_ca_sim_1/MATLAB Function4 ==
  data: tau output; rho input; loom output; rho_dot input; x4 output
function [tau, loom, x4] = fcn(rho, rho_dot)

loom = min(rho_dot/rho, 0);
if loom > -0.0001
    tau = 1000;
else
    tau = -1/loom;
end

x4 = 1/rho;

== matlab function multi_ca_sim_1/Subsystem1/MATLAB Function ==
  data: signal input; out output; bound1 input; bound2 input
function out = saturate(signal,bound1,bound2)
out = min(max(bound1,signal),bound2);

== matlab function multi_ca_sim_1/Subsystem1/MATLAB Function1 ==
  data: signal input; out output; bound1 input; bound2 input
function out = saturate(signal,bound1,bound2)
            out = min(max(bound1,signal),bound2);

== matlab function multi_ca_sim_1/Subsystem1/Subsystem5/Subsystem/MATLAB Function ==
  data: theta input; y output; delta input
function y = fcn(theta,delta)
if abs(theta-delta) <= 10^(-7)
    y=cos(theta);
else 
    y=(sin(theta)-sin(delta))/(theta-delta);
end

== matlab function multi_ca_sim_1/CA controller 3 ==
  data: u output; x1 input; x2 input; x3 input; x5 input; k input; r input; vr input; vo_max input; beta input; gamma input; omega input; ar input; x5 output; x2 output; x3 output; y output; alpha_1 output; alpha_2 output
function [u, x5, x2, x3,y, alpha_1, alpha_2]  = fcn(x1, x2 ,x3, x5, k, r, vr, vo_max,beta, gamma,omega, ar)


x6 = vr;

delta_t = ( pi - abs(wrapToPi_custom(x5-x2)))/(beta);

alpha_2 = -2*beta*omega*x1/(x6+vo_max);
alpha_1 = (k*x1^2 +  x6*max(0,-x3*sin(x5-x2)) -min(0, -ar*cos(x5-x2)) ) /(r + (x6 + vo_max )*delta_t);

 u =  sign_custom(wrapToPi_custom(x5-x2))*(gamma^2/beta*(x1^2  +alpha_1 ) +  alpha_2) + x3  ;
y = sign_custom(wrapToPi_custom(x5-x2));

if x1 >= 0
    u=0;
end

function y = sign_custom(x)

if x >= 0
    y = 1;
else
    y = -1;
end

function lambda = wrapTo2Pi_custom(lambda)
%wrapTo2Pi Wrap angle in radians to [0 2*pi]
%
%   lambdaWrapped = wrapTo2Pi(LAMBDA) wraps angles in LAMBDA, in radians,
%   to the interval [0 2*pi] such that zero maps to zero and 2*pi maps
%   to 2*pi. (In general, positive multiples of 2*pi map to 2*pi and
%   negative multiples of 2*pi map to zero.)
%
%   See also wrapToPi, wrapTo180, wrapTo360.

% Copyright 2007-2008 The MathWorks, Inc.

positiveInput = (lambda > 0);
lambda = mod(lambda, 2*pi);
lambda((lambda == 0) & positiveInput) = 2*pi;

function lambda = wrapToPi_custom(lambda)
%wrapToPi Wrap angle in radians to [-pi pi]
%
%   lambdaWrapped = wrapToPi(LAMBDA) wraps angles in LAMBDA, in radians,
%   to the interval [-pi pi] such that pi maps to pi and -pi maps to
%   -pi.  (In general, odd, positive multiples of pi map to pi and odd,
%   negative multiples of pi map to -pi.)
%
%   See also wrapTo2Pi, wrapTo180, wrapTo360.

% Copyright 2007-2008 The MathWorks, Inc.

q = (lambda < -pi) | (pi < lambda);
lambda(q) = wrapTo2Pi_custom(lambda(q) + pi) - pi;

== matlab function multi_ca_sim_1/MATLAB Function5 ==
  data: rho output; pos_vr input; lambda output; pos_obs input; psi_r input; psi_o input; vo input; vr input; dot_lambda output
function [rho, lambda, dot_lambda] = fcn(pos_vr, pos_obs, psi_r, psi_o, vo, vr)

lambda_vector = pos_obs-pos_vr;
rho = norm(lambda_vector,2);
lambda = atan2(lambda_vector(2), lambda_vector(1) );
dot_lambda = 1/rho*(vo*sin(psi_o - lambda) - vr*sin(psi_r - lambda));

== matlab function multi_ca_sim_1/MATLAB Function6 ==
  data: tau output; rho input; loom output; rho_dot input; x4 output
function [tau, loom, x4] = fcn(rho, rho_dot)

loom = min(rho_dot/rho, 0);
if loom > -0.0001
    tau = 1000;
else
    tau = -1/loom;
end

x4 = 1/rho;

== matlab function multi_ca_sim_1/Subsystem2/MATLAB Function ==
  data: signal input; out output; bound1 input; bound2 input
function out = saturate(signal,bound1,bound2)
out = min(max(bound1,signal),bound2);

== matlab function multi_ca_sim_1/Subsystem2/MATLAB Function1 ==
  data: signal input; out output; bound1 input; bound2 input
function out = saturate(signal,bound1,bound2)
            out = min(max(bound1,signal),bound2);

== matlab function multi_ca_sim_1/Subsystem2/Subsystem5/Subsystem/MATLAB Function ==
  data: theta input; y output; delta input
function y = fcn(theta,delta)
if abs(theta-delta) <= 10^(-7)
    y=cos(theta);
else 
    y=(sin(theta)-sin(delta))/(theta-delta);
end

== matlab function multi_ca_sim_1/vehicle1/MATLAB Function ==
  data: u input; y output; tan output
function [y,tan] = fcn(u)
theta = u/(1*1.5*4*pi);
y = [cos(theta) -sin(theta); sin(theta) cos(theta)]*[1*1.5*4*pi; 0];%*[5+6*pi*sin(pi/4)-6*pi*sin(1.2*pi/4)-0.5 15+6*pi*cos(pi/4)-6*pi*cos(1.2*pi/4)]';
tan = [-y(2); y(1)];

== matlab function multi_ca_sim_1/vehicle1/vehicle 1 ==
  data: speed_profile output; speed_target output; v_d_xi output; kappa output; t input; xi input; xi_dot input
function [speed_profile,speed_target, v_d_xi, kappa] = fcn(t,xi,xi_dot)
% vd=1.5;
% psi_d = t/pi/4 - pi/4;
% x_dot = 1.5*cos(psi_d);
% y_dot = 1.5*sin(psi_d);

%trajectory and speed profile
% x_dot = 0.9*1.5*cos(t/pi/4 - 1.2*pi/4);
% y_dot = 0.9*1.5*sin(t/pi/4 - 1.2*pi/4);
speed_profile=1*1.5;

%v_d(xi)
v_d_xi=1*1.5;
% v_d_xi=sqrt((0.9*1.5*cos(xi/pi/4 - 1.2*pi/4))^2+(0.9*1.5*sin(xi/pi/4 - 1.2*pi/4))^2);

%speed of target
speed_target = xi_dot*1*1.5;

%culvature
r=1*1.5*4*pi;
kappa=1/r;
